simulink model "simulation_wout_losses"  (R2022a)
settings: Solver=VariableStepAuto  StartTime=0.0  StopTime=0.5  FixedStep=1e-6  MaxStep=1e-6  RelTol=1e-3
libraries: spsCurrentMeasurementLib x7, spsSeriesRLCBranchLib x5, spsVoltageMeasurementLib x5, spsDCVoltageSourceLib x1, spsDiodeLib x1, spsIdealSwitchLib x1, spsVariableRatioTransformerLib x1, spspowerguiLib x1
settings Model: Creator=Arda  LastModifiedBy=isaer
settings DataIOCC: ReturnWorkspaceOutputs=off
settings ModelReferenceCC: EnableRefExpFcnMdlSchedulingChecks=off
settings RTWCC: Description=Generic Real-Time Target

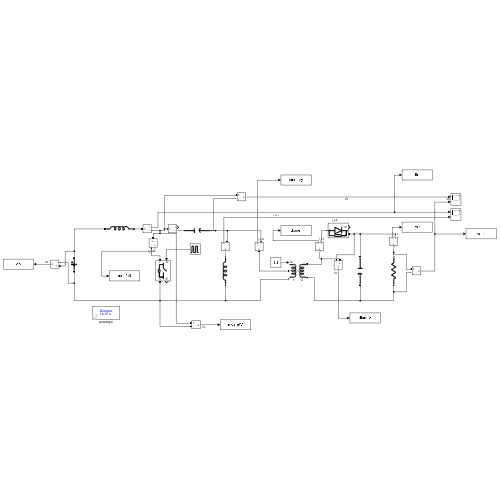
[thumbnail: Simulink's stored preview of the top-level diagram]
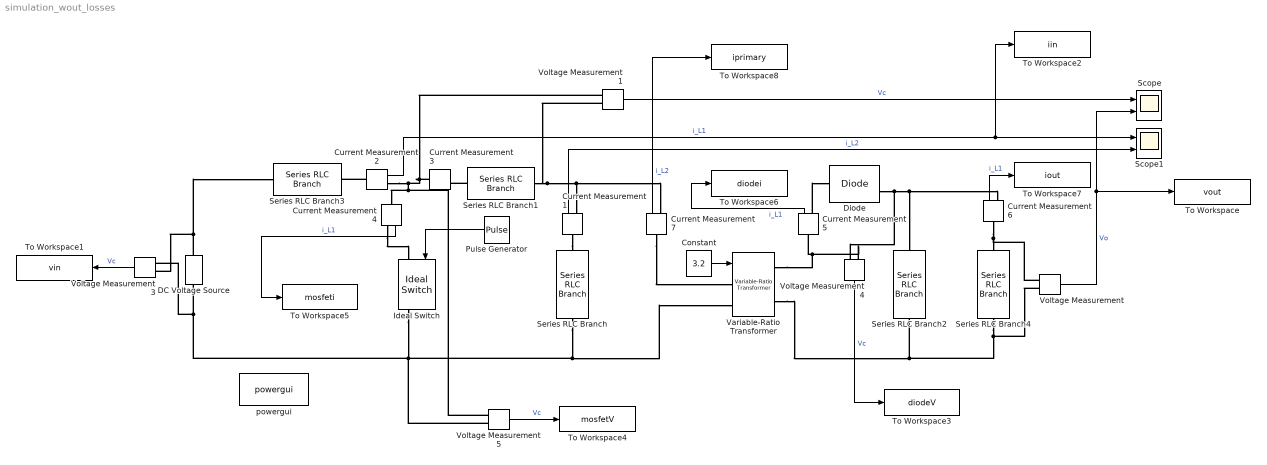
== system simulation_wout_losses ==
  Constant : Constant  Value=3.2
  Current Measurement{1..7} (7 alike) : spsCurrentMeasurementLib/Current Measurement  PhasorSimulation=off  OutputType=Complex  PSBequivalent=0
  DC Voltage Source : spsDCVoltageSourceLib/DC Voltage Source  Amplitude=12  Measurements=None
  Diode : spsDiodeLib/Diode  Ron=1e-3  Lon=0  Vf=0  IC=0  UseSnubber=0  Rs=500  Cs=250e-9  Measurements=on
  Ideal Switch : spsIdealSwitchLib/Ideal Switch  Ron=0.001  Lon=0  IC=0  Rs=1e5  Cs=inf  Measurements=on
  Pulse Generator : DiscretePulseGenerator  PulseType=Time based  Period=2e-5  PulseWidth=55.5
  Scope : Scope  NumInputPorts=2
  Scope1 : Scope  NumInputPorts=2
  Series RLC Branch : spsSeriesRLCBranchLib/Series RLC Branch  LConnTagsString=__new0  RConnTagsString=__new0  BranchType=L  Resistance=40e-3  Inductance=32.6e-6  SetiL0=off  InitialCurrent=0  Capacitance=1e-6  Setx0=off  InitialVoltage=0  Measurements=None
  Series RLC Branch1 : spsSeriesRLCBranchLib/Series RLC Branch  LConnTagsString=__new0  RConnTagsString=__new0  BranchType=C  Resistance=40e-3  Inductance=1e-3  SetiL0=off  InitialCurrent=0  Capacitance=10000e-3  Setx0=off  InitialVoltage=0  Measurements=None
  Series RLC Branch2 : spsSeriesRLCBranchLib/Series RLC Branch  LConnTagsString=__new0  RConnTagsString=__new0  BranchType=C  Resistance=40e-3  Inductance=1e-3  SetiL0=off  InitialCurrent=0  Capacitance=1e-3  Setx0=off  InitialVoltage=0  Measurements=None
  Series RLC Branch3 : spsSeriesRLCBranchLib/Series RLC Branch  LConnTagsString=__new0  RConnTagsString=__new0  BranchType=L  Resistance=40e-3  Inductance=32.6e-6  SetiL0=off  InitialCurrent=0  Capacitance=1e-6  Setx0=off  InitialVoltage=0  Measurements=None
  Series RLC Branch4 : spsSeriesRLCBranchLib/Series RLC Branch  LConnTagsString=__new0  RConnTagsString=__new0  BranchType=R  Resistance=48  Inductance=1e-3  SetiL0=off  InitialCurrent=0  Capacitance=10e-6  Setx0=off  InitialVoltage=0  Measurements=None
  To Workspace : ToWorkspace  VariableName=vout  SaveFormat=Timeseries  SampleTime=-1
  To Workspace1 : ToWorkspace  VariableName=vin  SaveFormat=Timeseries  SampleTime=-1
  To Workspace2 : ToWorkspace  VariableName=iin  SaveFormat=Timeseries  SampleTime=-1
  To Workspace3 : ToWorkspace  VariableName=diodeV  SaveFormat=Timeseries  SampleTime=-1
  To Workspace4 : ToWorkspace  VariableName=mosfetV  SaveFormat=Timeseries  SampleTime=-1
  To Workspace5 : ToWorkspace  VariableName=mosfeti  SaveFormat=Timeseries  SampleTime=-1
  To Workspace6 : ToWorkspace  VariableName=diodei  SaveFormat=Timeseries  SampleTime=-1
  To Workspace7 : ToWorkspace  VariableName=iout  SaveFormat=Timeseries  SampleTime=-1
  To Workspace8 : ToWorkspace  VariableName=iprimary  SaveFormat=Timeseries  SampleTime=-1
  Variable-Ratio Transformer : spsVariableRatioTransformerLib/Variable-Ratio Transformer
      settings: SourceProductBaseCode=PS
  Voltage Measurement{,1,3..5} (5 alike) : spsVoltageMeasurementLib/Voltage Measurement  PhasorSimulation=off  OutputType=Complex  PSBequivalent=0
  powergui : spspowerguiLib/powergui  Priority=1  SimulationMode=Discrete  SampleTime=1e-7  frequency=60  Iterations=50  frequencyindice=0  Pbase=100e6  ErrMax=1e-4  UnitsV=kV  UnitsW=MW  buscounter=0  FunctionMessages=off  echomessages=off  EnableUseOfTLC=off  CurrentSourceSwitches=off  DisableSnubberDevices=off  DisableRonSwitches=off  DisableVfSwitches=off  DisplayEquations=off  AutomaticDiscreteSolvers=off  SolverType=Tustin/Backward Euler (TBE)  Interpol=off  ExternalGateDelay=off  methode=off  Ts=100  x0status=blocks  SPID=on  SwTol=0  HookPort=off  NonlinearTolerance=1e-4  nMaxIteration=100  ContinueOnMaxIteration=off  RestoreLinks=warning  ResistiveCurrentMeasurement=off  Frange=[0:2:500]  Ylog=off  Xlog=on  ShowGrid=off  save=off  variable=ZData  structure=0  ZoomFFT=off  StartTime=0.0  cycles=1  DisplayStyle=1  fundamental=60  FreqAxis=off  MaxFrequency=1000  frequencyindicesteady=1  RmsSteady=1  display=off
  wires:
  Pulse Generator/1 -> Ideal Switch/1
  Voltage Measurement1/1 -> Scope/1  "Vc"
  Voltage Measurement/1 -> To Workspace/1, Scope/2  "Vo"
  Current Measurement2/1 -> To Workspace2/1, Scope1/1  "i_L1"
  Current Measurement1/1 -> Scope1/2  "i_L2"
  Constant/1 -> Variable-Ratio Transformer/1
  Voltage Measurement3/1 -> To Workspace1/1  "Vc"
  Voltage Measurement4/1 -> To Workspace3/1  "Vc"
  Voltage Measurement5/1 -> To Workspace4/1  "Vc"
  Current Measurement4/1 -> To Workspace5/1  "i_L1"
  Current Measurement5/1 -> To Workspace6/1  "i_L1"
  Current Measurement6/1 -> To Workspace7/1  "i_L1"
  Current Measurement7/1 -> To Workspace8/1  "i_L2"
  connections:
  Current Measurement1/LConn1 -- Series RLC Branch/RConn1
  Current Measurement2/LConn1 -- Series RLC Branch3/RConn1
  DC Voltage Source/RConn1 -- Series RLC Branch3/LConn1 -- Voltage Measurement3/LConn1
  Current Measurement2/RConn1 -- Voltage Measurement5/LConn1 -- Current Measurement4/LConn1 -- Current Measurement3/LConn1 -- Voltage Measurement1/LConn1
  Current Measurement7/LConn1 -- Variable-Ratio Transformer/LConn1
  Diode/RConn1 -- Voltage Measurement4/LConn2 -- Series RLC Branch2/LConn1 -- Current Measurement6/RConn1
  Voltage Measurement/LConn2 -- Series RLC Branch4/RConn1 -- Variable-Ratio Transformer/RConn2 -- Series RLC Branch2/RConn1
  Variable-Ratio Transformer/RConn1 -- Voltage Measurement4/LConn1 -- Current Measurement5/LConn1
  Ideal Switch/RConn1 -- Voltage Measurement5/LConn2 -- Series RLC Branch/LConn1 -- Variable-Ratio Transformer/LConn2 -- Voltage Measurement3/LConn2 -- DC Voltage Source/LConn1
  Series RLC Branch1/LConn1 -- Current Measurement3/RConn1
  Current Measurement4/RConn1 -- Ideal Switch/LConn1
  Current Measurement5/RConn1 -- Diode/LConn1
  Current Measurement6/LConn1 -- Voltage Measurement/LConn1 -- Series RLC Branch4/LConn1
  Voltage Measurement1/LConn2 -- Series RLC Branch1/RConn1 -- Current Measurement7/RConn1 -- Current Measurement1/RConn1
